simulink library "limblab"  (Simulink 6.6)
undefined symbols (not defined in the file or in its folder): dfilt
libraries: simulink x20, xpclib x10, xpcnilib x5, limblab x5, dsparch4 x4, xpcmeasurementcomputinglib x2, dspmtrx3 x1, simulink_extras x1
settings Model: Creator=limblab  LastModifiedBy=limblab

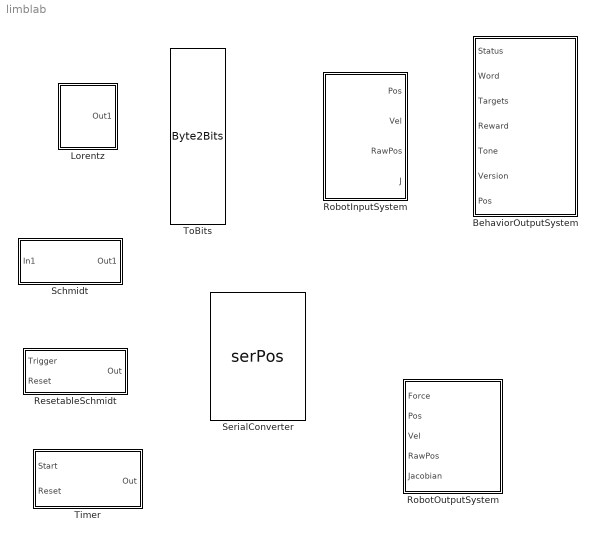
== system limblab ==
  BehaviorOutputSystem : Subsystem  TreatAsAtomicUnit=on  mask{RewardPulse=0}
      mask prompts: RewardPulse "Reward Pulse"
      mask Display:
      | port_label('input',1,'Status')
      | port_label('input',2,'Word')
      | port_label('input',3,'Targets')
      | port_label('input',4,'Reward')
      | port_label('input',5,'Tone')
      | port_label('input',6,'Version')
      | port_label('input',7,'Position')
  Lorentz : Subsystem  TreatAsAtomicUnit=on  mask(Lorentz attractor){y0=.1}
      mask prompts: y0 "Initial Condition"
      mask help: Creats chaotic oscelations using a lorentz attractor algorithm.
      mask Help:
      | Creats chaotic oscelations using a lorentz attractor algorithm.
      | 
      | This particular oscilator has the parameters:
      | rho = 28
      | beta = 8/3
      | sigma = 10
      | 
      | The initial condition y0 can be specified as a parameter.
      | 
      | Other initial conditions (x0 and z0) are 0.1.
      mask Display: port_label('output', 1, 'Out')
  ResetableSchmidt : Subsystem  TreatAsAtomicUnit=on  mask{Time=3}
  RobotInputSystem : Subsystem  TreatAsAtomicUnit=on  mask{ShOffset=0, ElOffset=0, XOffset=2, YOffset=-36, Ang=0}
      mask prompts: ShOffset "Shoulder Offset"; ElOffset "Elbow Offset"; XOffset "X Offset"; YOffset "Y Offset"; Ang "Cursor Rotation"
      mask Display:
      | port_label('output',1,'Position')
      | port_label('output',2,'Velocity')
      | port_label('output',3,'Raw Position')
      | port_label('output',4,'Jacobian')
  RobotOutputSystem : Subsystem  TreatAsAtomicUnit=on  mask{RecFlag=off, XHighLimit=25, XLowLimit=-30, YHighLimit=-46, YLowLimit=-22}
      mask prompts: RecFlag "Recenter Handle"; XHighLimit "X Upper Limit"; XLowLimit "X Lower Limit"; YHighLimit "Y Upper Limit"; YLowLimit "Y Lower Limit"
      mask Display:
      | port_label('input', 1, 'Force')
      | port_label('input', 2, 'Position')
      | port_label('input', 3, 'Velocity')
      | port_label('input', 4, 'Raw Position')
      | port_label('input', 5, 'Jacobian')
  Schmidt : Subsystem  TreatAsAtomicUnit=on  mask(Schmidt Trigger){Time=.3}
      mask help: Creates an output pulse of the specified time in seconds when trig goes high
      mask Help: Creates an output pulse of the specified time in seconds when trig goes high
      mask Display:
      | port_label('output',1,'out')
      | port_label('input',1,'trig')
      | fprintf('t = %.2f',Time)
  SerialConverter : S-Function  FunctionName=serPos
      mask Display:
      | port_label('output', 1, 'Byte Out')
      | port_label('input', 1, 'index')
      | port_label('input', 2, 'sh')
      | port_label('input', 3, 'el')
  Timer : Subsystem  TreatAsAtomicUnit=on  mask{Time=.1}
      mask prompts: Time "Timeout"
      mask Display:
      | port_label('output',1,'out')
      | port_label('input',1,'start')
      | port_label('input',2,'reset')
      | fprintf('t = %.2f',Time)
  ToBits : S-Function  FunctionName=Byte2Bits
      mask Display:
      | port_label('input', 1, 'u')
      | port_label('output', 1, 'y0')
      | port_label('output', 2, 'y1')
      | port_label('output', 3, 'y2')
      | port_label('output', 4, 'y3')
      | port_label('output', 5, 'y4')
      | port_label('output', 6, 'y5')
      | port_label('output', 7, 'y6')
      | port_label('output', 8, 'y7')

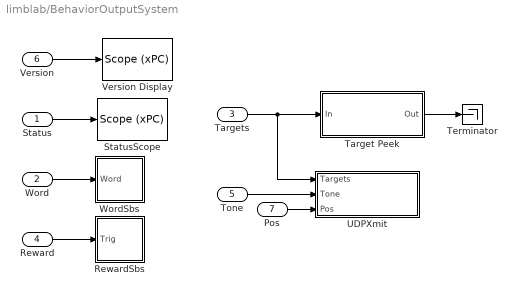
== system limblab/BehaviorOutputSystem ==
  Status : Inport
  Word : Inport  Port=2
  Targets : Inport  Port=3
  Reward : Inport  Port=4
  Tone : Inport  Port=5
  Version : Inport  Port=6
  Pos : Inport  Port=7
  RewardSbs : Subsystem
  StatusScope : xpclib/Misc./Scope (xPC)   SystemSampleTime=-1  scopeno=2  scopetype=Target  autostart=on  viewmode=Numerical  formatstr='%6.0f state,%6.0f rewards,%6.0f aborts,%6.0f fails,%6.0f incompl'  grid=on  ylimits=[-10,10]  nosamples=10  noprepostsamples=0  interleave=10  triggermode=FreeRun  triggersignal=1  triggerlevel=0.0  triggerslope=Either  triggerscope=1  triggersample=0  filename=data.dat  mode=Lazy  writesize=512  autorestart=off
  Target Peek : Subsystem
  Terminator : Terminator
  UDPXmit : Subsystem
  Version Display : xpclib/Misc./Scope (xPC)   SystemSampleTime=-1  scopeno=3  scopetype=Target  autostart=on  viewmode=Numerical  formatstr='%6.0f major,%6.0f minor,%6.0f revision,%6.0f build'  grid=on  ylimits=[-10,10]  nosamples=10  noprepostsamples=0  interleave=10  triggermode=FreeRun  triggersignal=1  triggerlevel=0.0  triggerslope=Either  triggerscope=1  triggersample=0  filename=data.dat  mode=Lazy  writesize=512  autorestart=off
  WordSbs : Subsystem
  wires:
  Status/1 -> StatusScope/1
  Word/1 -> WordSbs/1(Word)
  Targets/1 -> Target Peek/1(In), UDPXmit/1(Targets)
  Reward/1 -> RewardSbs/1(Trig)
  Target Peek/1(Out) -> Terminator/1
  Version/1 -> Version Display/1
  Pos/1 -> UDPXmit/3(Pos)
  Tone/1 -> UDPXmit/2(Tone)

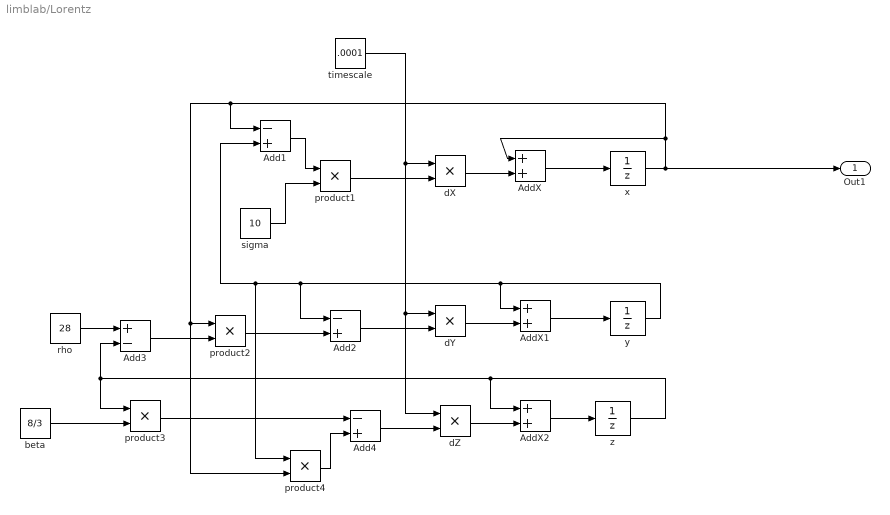
== system limblab/Lorentz ==
  Add1 : Sum  Inputs=-+  OutScaling=2^-10
  Add2 : Sum  Inputs=-+  OutScaling=2^-10
  Add3 : Sum  Inputs=+-  OutScaling=2^-10
  Add4 : Sum  Inputs=-+  OutScaling=2^-10
  AddX : Sum  OutScaling=2^-10
  AddX1 : Sum  OutScaling=2^-10
  AddX2 : Sum  OutScaling=2^-10
  beta : Constant  Value=8/3
  dX : Product  RndMeth=Zero
  dY : Product  RndMeth=Zero
  dZ : Product  RndMeth=Zero
  product{1..4} (4 alike) : Product  RndMeth=Zero
  rho : Constant  Value=28
  sigma : Constant  Value=10
  timescale : Constant  Value=.0001
  x : UnitDelay  X0=.1  SampleTime=.001
  y : UnitDelay  X0=y0  SampleTime=.001
  z : UnitDelay  X0=.1  SampleTime=.001
  Out1 : Outport
  wires:
  AddX/1 -> x/1
  AddX1/1 -> y/1
  AddX2/1 -> z/1
  y/1 -> AddX1/1, Add2/1, Add1/2, product4/1
  z/1 -> AddX2/1, Add3/2, product3/1
  x/1 -> Out1/1, AddX/1, Add1/1, product2/1, product4/2
  dX/1 -> AddX/2
  dY/1 -> AddX1/2
  dZ/1 -> AddX2/2
  timescale/1 -> dX/1, dY/1, dZ/1
  sigma/1 -> product1/2
  product1/1 -> dX/2
  Add1/1 -> product1/1
  Add2/1 -> dY/2
  product2/1 -> Add2/2
  Add3/1 -> product2/2
  rho/1 -> Add3/1
  beta/1 -> product3/2
  product3/1 -> Add4/1
  product4/1 -> Add4/2
  Add4/1 -> dZ/2

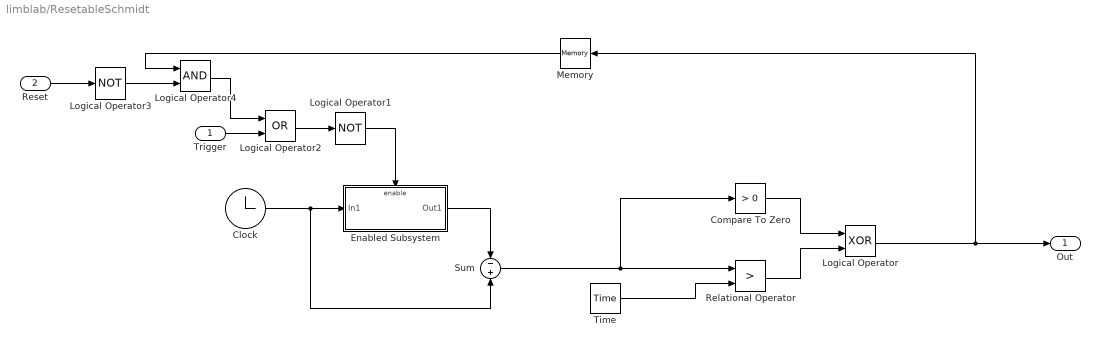
== system limblab/ResetableSchmidt ==
  Trigger : Inport
  Reset : Inport  Port=2
  Clock : Clock
  Compare To Zero : simulink/Logic and Bit Operations/Compare To Zero  SystemSampleTime=-1  relop=>  LogicOutDataTypeMode=uint8  ZeroCross=off
  Enabled Subsystem : Subsystem  TreatAsAtomicUnit=on
  Logical Operator : Logic  Operator=XOR  AllPortsSameDT=off  OutDataTypeMode=Boolean  SampleTime=.001
  Logical Operator1 : Logic  Operator=NOT  AllPortsSameDT=off  OutDataTypeMode=Boolean
  Logical Operator2 : Logic  Operator=OR  AllPortsSameDT=off  OutDataTypeMode=Boolean  SampleTime=.001
  Logical Operator3 : Logic  Operator=NOT  AllPortsSameDT=off  OutDataTypeMode=Boolean
  Logical Operator4 : Logic  AllPortsSameDT=off  OutDataTypeMode=Boolean  SampleTime=.001
  Memory : Memory  Orientation=left
  Relational Operator : RelationalOperator  Operator=>  LogicOutDataTypeMode=Boolean
  Sum : Sum  Inputs=-+
  Time : Constant  Value=Time
  Out : Outport
  wires:
  Logical Operator2/1 -> Logical Operator1/1
  Trigger/1 -> Logical Operator2/2
  Logical Operator/1 -> Memory/1, Out/1
  Logical Operator1/1 -> Enabled Subsystem/Enable
  Relational Operator/1 -> Logical Operator/2
  Compare To Zero/1 -> Logical Operator/1
  Time/1 -> Relational Operator/2
  Sum/1 -> Relational Operator/1, Compare To Zero/1
  Enabled Subsystem/1(Out1) -> Sum/1
  Clock/1 -> Sum/2, Enabled Subsystem/1(In1)
  Reset/1 -> Logical Operator3/1
  Logical Operator3/1 -> Logical Operator4/2
  Logical Operator4/1 -> Logical Operator2/1
  Memory/1 -> Logical Operator4/1

== system limblab/RobotInputSystem ==
  Matrix Concatenation1 : Concatenate  Mode=Vector
  Velocity Calculation : Subsystem
  XY Position Subsystem : Subsystem
  Xpos : xpclib/Misc./Scope (xPC)   SystemSampleTime=-1  scopeno=1  scopetype=Target  autostart=on  viewmode=Numerical  formatstr='%15.2f X,%15.2f Y,%15.2f dX,%15.2f dY,%15.2f Fx,%15.2f Fy'  grid=on  ylimits=[-10,10]  nosamples=10  noprepostsamples=0  interleave=10  triggermode=FreeRun  triggersignal=1  triggerlevel=0.0  triggerslope=Either  triggerscope=1  triggersample=0  filename=data.dat  mode=Lazy  writesize=512  autorestart=off
  Pos : Outport
  Vel : Outport  Port=2
  RawPos : Outport  Port=3
  J : Outport  Port=4
  wires:
  Velocity Calculation/1(Vel) -> Matrix Concatenation1/2, Vel/1
  XY Position Subsystem/1(Pos) -> Velocity Calculation/1(Pos), Matrix Concatenation1/1, Pos/1
  Matrix Concatenation1/1 -> Xpos/1
  XY Position Subsystem/3(RawPos) -> RawPos/1
  XY Position Subsystem/2(J) -> Velocity Calculation/2(J), J/1

== system limblab/RobotOutputSystem ==
  Force : Inport
  Pos : Inport  Port=2
  Vel : Inport  Port=3
  RawPos : Inport  Port=4
  Jacobian : Inport  Port=5
  BoundingBox : Subsystem
  Motor Control : Subsystem
  Recentering Subsystem : Subsystem
  wires:
  Recentering Subsystem/2(toSwitch) -> Motor Control/3(Switch)
  Recentering Subsystem/1(Forces) -> Motor Control/2(Recenter/Arrest Force)
  BoundingBox/1(Out) -> Recentering Subsystem/3(OutsideBox)
  Force/1 -> Motor Control/1(DefaultForce)
  Jacobian/1 -> Motor Control/4(Jacobian)
  Vel/1 -> Recentering Subsystem/1(Vel)
  Pos/1 -> Recentering Subsystem/2(Pos)
  RawPos/1 -> BoundingBox/1(RawPos)

== system limblab/Schmidt ==
  In1 : Inport
  Clock : Clock
  Compare To Zero : simulink/Logic and Bit Operations/Compare To Zero  SystemSampleTime=-1  relop=>  LogicOutDataTypeMode=uint8  ZeroCross=off
  Enabled Subsystem : Subsystem  TreatAsAtomicUnit=on
  Logical Operator : Logic  Operator=XOR  AllPortsSameDT=off  OutDataTypeMode=Boolean  SampleTime=.001
  Logical Operator1 : Logic  Operator=NOT  AllPortsSameDT=off  OutDataTypeMode=Boolean
  Logical Operator2 : Logic  Operator=OR  AllPortsSameDT=off  OutDataTypeMode=Boolean  SampleTime=.001
  Memory : Memory  Orientation=left
  Relational Operator : RelationalOperator  Operator=>  LogicOutDataTypeMode=Boolean
  Sum : Sum  Inputs=-+
  Time : Constant  Value=Time
  Out1 : Outport
  wires:
  Clock/1 -> Enabled Subsystem/1(In1), Sum/2
  Enabled Subsystem/1(Out1) -> Sum/1
  Sum/1 -> Compare To Zero/1, Relational Operator/1
  Time/1 -> Relational Operator/2
  Compare To Zero/1 -> Logical Operator/1
  Relational Operator/1 -> Logical Operator/2
  Logical Operator1/1 -> Enabled Subsystem/Enable
  Logical Operator/1 -> Out1/1, Memory/1
  In1/1 -> Logical Operator2/2
  Logical Operator2/1 -> Logical Operator1/1
  Memory/1 -> Logical Operator2/1

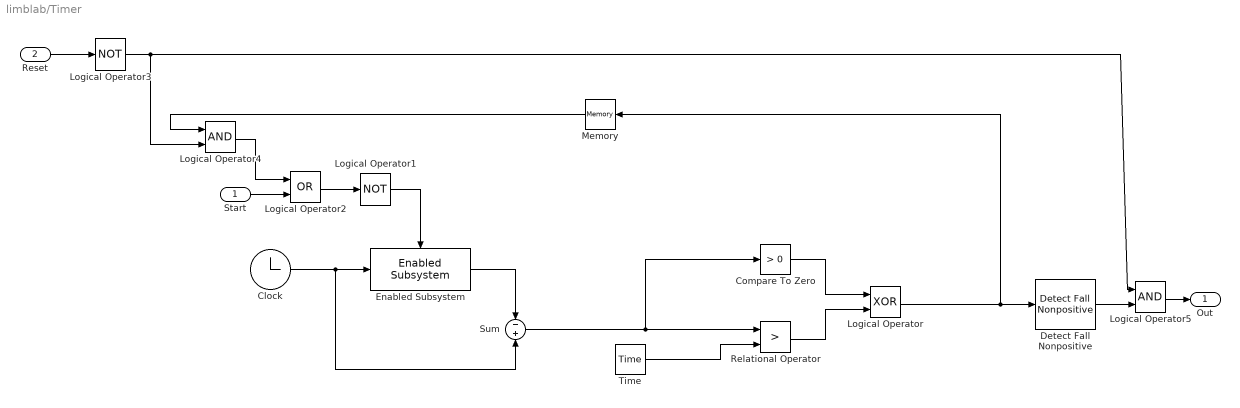
== system limblab/Timer ==
  Start : Inport
  Reset : Inport  Port=2
  Clock : Clock
  Compare To Zero : simulink/Logic and Bit Operations/Compare To Zero  SystemSampleTime=-1  relop=>  LogicOutDataTypeMode=uint8  ZeroCross=off
  Detect Fall Nonpositive : simulink/Logic and Bit Operations/Detect Fall Nonpositive  SystemSampleTime=-1  vinit=0
  Enabled Subsystem : limblab/ResetableSchmidt/Enabled Subsystem  SystemSampleTime=-1
  Logical Operator : Logic  Operator=XOR  AllPortsSameDT=off  OutDataTypeMode=Boolean  SampleTime=.001
  Logical Operator1 : Logic  Operator=NOT  AllPortsSameDT=off  OutDataTypeMode=Boolean
  Logical Operator2 : Logic  Operator=OR  AllPortsSameDT=off  OutDataTypeMode=Boolean  SampleTime=.001
  Logical Operator3 : Logic  Operator=NOT  AllPortsSameDT=off  OutDataTypeMode=Boolean
  Logical Operator4 : Logic  AllPortsSameDT=off  OutDataTypeMode=Boolean  SampleTime=.001
  Logical Operator5 : Logic  AllPortsSameDT=off  OutDataTypeMode=Boolean  SampleTime=.001
  Memory : Memory  Orientation=left
  Relational Operator : RelationalOperator  Operator=>  LogicOutDataTypeMode=Boolean
  Sum : Sum  Inputs=-+
  Time : Constant  Value=Time
  Out : Outport
  wires:
  Memory/1 -> Logical Operator4/1
  Logical Operator4/1 -> Logical Operator2/1
  Logical Operator3/1 -> Logical Operator5/1, Logical Operator4/2
  Reset/1 -> Logical Operator3/1
  Clock/1 -> Sum/2, Enabled Subsystem/1
  Enabled Subsystem/1 -> Sum/1
  Sum/1 -> Relational Operator/1, Compare To Zero/1
  Time/1 -> Relational Operator/2
  Compare To Zero/1 -> Logical Operator/1
  Relational Operator/1 -> Logical Operator/2
  Logical Operator1/1 -> Enabled Subsystem/Enable
  Logical Operator/1 -> Memory/1, Detect Fall Nonpositive/1
  Start/1 -> Logical Operator2/2
  Logical Operator2/1 -> Logical Operator1/1
  Detect Fall Nonpositive/1 -> Logical Operator5/2
  Logical Operator5/1 -> Out/1

== system limblab/BehaviorOutputSystem/RewardSbs ==
  Trig : Inport
  Data Type Conversion : DataTypeConversion
  Memory1 : Memory
  Schmidt1 : Subsystem  mask(Schmidt Trigger){Time=RewardPulse}
      mask help: Creates an output pulse of the specified time in seconds when trig goes high
      mask Help: Creates an output pulse of the specified time in seconds when trig goes high
      mask Display:
      | port_label('output',1,'out')
      | port_label('input',1,'trig')
      | fprintf('t = %.2f',Time)
  tag scope: Reward=global
  wires:
  Trig/1 -> Schmidt1/1(In1)
  Schmidt1/1(Out1) -> Memory1/1
  Memory1/1 -> Data Type Conversion/1
  Data Type Conversion/1 -> [Reward]

== system limblab/BehaviorOutputSystem/Target Peek ==
  In : Inport
  Add : Sum  OutScaling=2^-10
  Add1 : Sum  OutScaling=2^-10
  Demux : Demux  Outputs=10
  Gain : Gain  Gain=.5
  Gain1 : Gain  Gain=.5
  Mux : Mux  Inputs=3
  Terminator{,1..4} (5 alike) : Terminator
  Out : Outport
  wires:
  In/1 -> Demux/1
  Mux/1 -> Out/1
  Demux/1 -> Mux/1
  Add/1 -> Gain/1
  Add1/1 -> Gain1/1
  Gain1/1 -> Mux/3
  Demux/7 -> Terminator/1
  Demux/8 -> Terminator1/1
  Demux/9 -> Terminator2/1
  Demux/10 -> Terminator3/1
  Demux/2 -> Add/1
  Demux/4 -> Add/2
  Demux/3 -> Add1/1
  Demux/5 -> Add1/2
  Demux/6 -> Terminator4/1
  Gain/1 -> Mux/2

== system limblab/BehaviorOutputSystem/UDPXmit ==
  Targets : Inport
  Tone : Inport  Port=2
  Pos : Inport  Port=3
  Demux : Demux  Outputs=10
  Demux1 : Demux  Outputs=2
  Demux2 : Demux  Outputs=2
  Pack : xpclib/UDP/Pack  datatypes={'double', 'double','double','double','double','double','double','double','double','double','double','double','double','double'}  byteAlign=1
  Rate Transition : RateTransition
  Send : xpclib/UDP/Send  ipAddress=192.168.0.2  ipPort=25000  localPort=-1  sampletime=.02
  wires:
  Rate Transition/1 -> Send/1
  Pack/1 -> Rate Transition/1
  Demux/10 -> Pack/12
  Demux/9 -> Pack/11
  Demux/8 -> Pack/10
  Demux/7 -> Pack/9
  Demux/6 -> Pack/8
  Demux/5 -> Pack/7
  Demux/4 -> Pack/6
  Demux/3 -> Pack/5
  Demux/2 -> Pack/4
  Demux/1 -> Pack/3
  Demux1/1 -> Pack/1
  Demux1/2 -> Pack/2
  Demux2/1 -> Pack/13
  Demux2/2 -> Pack/14
  Tone/1 -> Demux2/1
  Targets/1 -> Demux/1
  Pos/1 -> Demux1/1

== system limblab/BehaviorOutputSystem/WordSbs ==
  Word : Inport
  tag scope: Word=global
  wires:
  Word/1 -> [Word]

== system limblab/ResetableSchmidt/Enabled Subsystem ==
  In1 : Inport
  Enable : EnablePort
  Out1 : Outport
  wires:
  In1/1 -> Out1/1

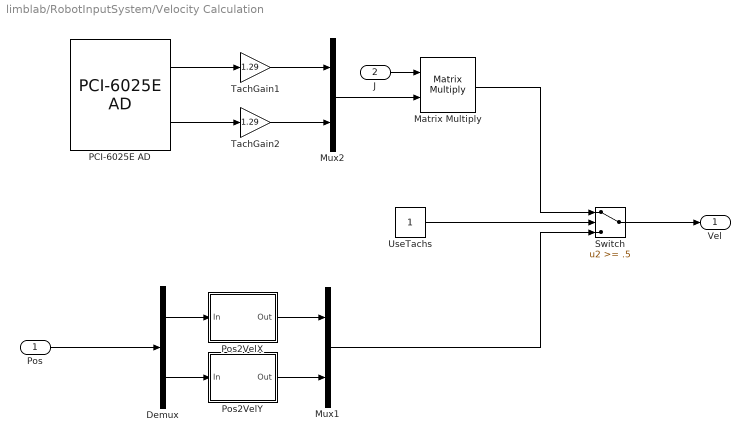
== system limblab/RobotInputSystem/Velocity Calculation ==
  Pos : Inport
  J : Inport  Port=2
  Demux : Demux  Outputs=2
  Matrix Multiply : Product  Multiplication=Matrix(*)
  Mux1 : Mux  Inputs=2
  Mux2 : Mux  Inputs=2
  PCI-6025E AD : xpcnilib/A//D/PCI-6025E AD  channel=[1,2]  range=[-10,-10]  coupling=[0,0]  sampletime=0.001  slot=-1
  Pos2VelX : Subsystem
  Pos2VelY : Subsystem
  Switch : Switch  Threshold=.5
  TachGain1 : Gain  Gain=1.29
  TachGain2 : Gain  Gain=1.29
  UseTachs : Constant
  Vel : Outport
  wires:
  Pos2VelX/1(Out) -> Mux1/1
  Pos2VelY/1(Out) -> Mux1/2
  Demux/1 -> Pos2VelX/1(In)
  Demux/2 -> Pos2VelY/1(In)
  Pos/1 -> Demux/1
  UseTachs/1 -> Switch/2
  PCI-6025E AD/1 -> TachGain1/1
  PCI-6025E AD/2 -> TachGain2/1
  TachGain1/1 -> Mux2/1
  TachGain2/1 -> Mux2/2
  J/1 -> Matrix Multiply/1
  Mux2/1 -> Matrix Multiply/2
  Switch/1 -> Vel/1
  Mux1/1 -> Switch/3
  Matrix Multiply/1 -> Switch/1

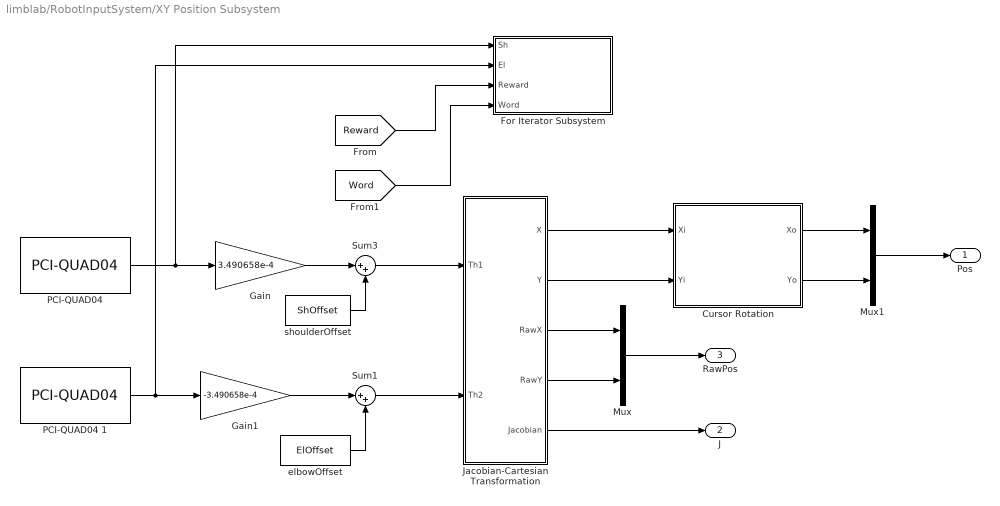
== system limblab/RobotInputSystem/XY Position Subsystem ==
  Cursor Rotation : Subsystem
  For Iterator Subsystem : Subsystem  TreatAsAtomicUnit=on
  Gain : Gain  Gain=3.490658e-4
  Gain1 : Gain  Gain=-3.490658e-4
  Jacobian-Cartesian Transformation : Subsystem
  Mux : Mux  Inputs=2
  Mux1 : Mux  Inputs=2
  "PCI-QUAD04 " : xpcmeasurementcomputinglib/Incremental Encoder/PCI-QUAD04   channel=1  resetmode=on  polarity=Positive Index  mode=Normal  limit=0  range=-2^23...+2^23-1  speed=1x  prescale=0  ts=0.001  convbaseaddr=-1
  PCI-QUAD04 1 : xpcmeasurementcomputinglib/Incremental Encoder/PCI-QUAD04   channel=2  resetmode=on  polarity=Positive Index  mode=Normal  limit=0  range=-2^23...+2^23-1  speed=1x  prescale=0  ts=0.001  convbaseaddr=-1
  Sum1 : Sum  Inputs=|++  SaturateOnIntegerOverflow=on  InputSameDT=on
  Sum3 : Sum  Inputs=|++  SaturateOnIntegerOverflow=on  InputSameDT=on
  elbowOffset : Constant  Value=ElOffset
  shoulderOffset : Constant  Value=ShOffset
  Pos : Outport
  J : Outport  Port=2
  RawPos : Outport  Port=3
  wires:
  PCI-QUAD04 1/1 -> For Iterator Subsystem/2("El "), Gain1/1
  "PCI-QUAD04 "/1 -> For Iterator Subsystem/1(Sh), Gain/1
  Gain/1 -> Sum3/1
  Sum3/1 -> Jacobian-Cartesian Transformation/1(Th1)
  shoulderOffset/1 -> Sum3/2
  Gain1/1 -> Sum1/1
  elbowOffset/1 -> Sum1/2
  Sum1/1 -> Jacobian-Cartesian Transformation/2(Th2)
  Jacobian-Cartesian Transformation/1(X) -> Cursor Rotation/1(Xi)
  Jacobian-Cartesian Transformation/2(Y) -> Cursor Rotation/2(Yi)
  Cursor Rotation/1(Xo) -> Mux1/1
  Cursor Rotation/2(Yo) -> Mux1/2
  Jacobian-Cartesian Transformation/3(RawX) -> Mux/1
  Jacobian-Cartesian Transformation/4(RawY) -> Mux/2
  [Reward] -> For Iterator Subsystem/3(Reward)
  Jacobian-Cartesian Transformation/5(Jacobian) -> J/1
  Mux/1 -> RawPos/1
  Mux1/1 -> Pos/1
  [Word] -> For Iterator Subsystem/4(Word)

== system limblab/RobotOutputSystem/BoundingBox ==
  note: 1: if [X Y] is outside
      | bounding box
      | 0: otherwise
  RawPos : Inport
  Demux : Demux  Outputs=2
  Logical Operator : Logic  Operator=OR  Inputs=4  AllPortsSameDT=off  OutDataTypeMode=Boolean
  Relational Operator : RelationalOperator  Operator=<  LogicOutDataTypeMode=Boolean
  Relational Operator1 : RelationalOperator  Operator=>  LogicOutDataTypeMode=Boolean
  Relational Operator2 : RelationalOperator  Operator=<  LogicOutDataTypeMode=Boolean
  Relational Operator3 : RelationalOperator  Operator=>  LogicOutDataTypeMode=Boolean
  XHighLimit : Constant  Value=XHighLimit
  XLowLimit : Constant  Value=XLowLimit
  YHighLimit : Constant  Value=YHighLimit
  YLowLimit : Constant  Value=YLowLimit
  Out : Outport
  wires:
  XLowLimit/1 -> Relational Operator/2
  XHighLimit/1 -> Relational Operator1/2
  YHighLimit/1 -> Relational Operator2/2
  YLowLimit/1 -> Relational Operator3/2
  Relational Operator/1 -> Logical Operator/1
  Relational Operator1/1 -> Logical Operator/2
  Relational Operator2/1 -> Logical Operator/3
  Relational Operator3/1 -> Logical Operator/4
  Logical Operator/1 -> Out/1
  RawPos/1 -> Demux/1
  Demux/1 -> Relational Operator/1, Relational Operator1/1
  Demux/2 -> Relational Operator2/1, Relational Operator3/1

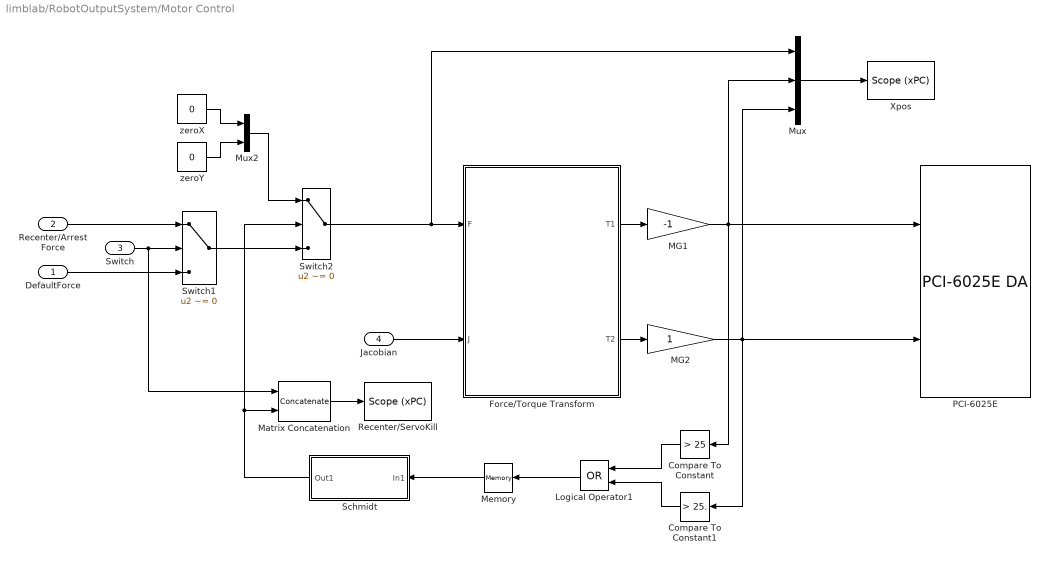
== system limblab/RobotOutputSystem/Motor Control ==
  DefaultForce : Inport
  Recenter/Arrest Force : Inport  Port=2
  Switch : Inport  Port=3
  Jacobian : Inport  Port=4
  Compare To Constant : simulink/Logic and Bit Operations/Compare To Constant  Orientation=left  SystemSampleTime=-1  relop=>  const=25  LogicOutDataTypeMode=uint8  ZeroCross=off
  Compare To Constant1 : simulink/Logic and Bit Operations/Compare To Constant  Orientation=left  SystemSampleTime=-1  relop=>  const=25.  LogicOutDataTypeMode=uint8  ZeroCross=off
  Force/Torque Transform : Subsystem  TreatAsAtomicUnit=on
  Logical Operator1 : Logic  Orientation=left  Operator=OR  AllPortsSameDT=off  OutDataTypeMode=Boolean
  MG1 : Gain  Gain=-1
  MG2 : Gain
  Matrix Concatenation : Concatenate  Mode=Vector
  Memory : Memory  Orientation=left
  Mux : Mux  Inputs=3
  Mux2 : Mux  Inputs=2
  "PCI-6025E " : xpcnilib/D//A/PCI-6025E DA  channel=[1 2]  reset=[1 1]  initValue=[0 0]  sampletime=0.001  slot=-1
  Recenter/ServoKill : xpclib/Misc./Scope (xPC)   SystemSampleTime=-1  scopeno=5  scopetype=Target  autostart=on  viewmode=Numerical  formatstr='%6.0f Control,%6.0f ServoKill'  grid=on  ylimits=[-10,10]  nosamples=10  noprepostsamples=0  interleave=10  triggermode=FreeRun  triggersignal=1  triggerlevel=0.0  triggerslope=Either  triggerscope=1  triggersample=0  filename=data.dat  mode=Lazy  writesize=512  autorestart=off
  Schmidt : Subsystem  Orientation=left  mask(Schmidt Trigger){Time=3}
      mask help: Creates an output pulse of the specified time in seconds when trig goes high
      mask Help: Creates an output pulse of the specified time in seconds when trig goes high
      mask Display:
      | port_label('output',1,'out')
      | port_label('input',1,'trig')
      | fprintf('t = %d',Time)
  Switch1 : Switch  Criteria=u2 ~= 0  ZeroCross=off
  Switch2 : Switch  Criteria=u2 ~= 0  ZeroCross=off
  Xpos : xpclib/Misc./Scope (xPC)   SystemSampleTime=-1  scopeno=6  scopetype=Target  autostart=on  viewmode=Numerical  formatstr='%15.2f Fx,%15.2f Fy,%15.2f T1,%15.2f T2'  grid=on  ylimits=[-10,10]  nosamples=10  noprepostsamples=0  interleave=10  triggermode=FreeRun  triggersignal=1  triggerlevel=0.0  triggerslope=Either  triggerscope=1  triggersample=0  filename=data.dat  mode=Lazy  writesize=512  autorestart=off
  zeroX : Constant  Value=0
  zeroY : Constant  Value=0
  wires:
  MG1/1 -> Compare To Constant/1, Mux/2, "PCI-6025E "/1
  MG2/1 -> Compare To Constant1/1, Mux/3, "PCI-6025E "/2
  Force/Torque Transform/1(T1) -> MG1/1
  Force/Torque Transform/2(T2) -> MG2/1
  zeroX/1 -> Mux2/1
  zeroY/1 -> Mux2/2
  Mux2/1 -> Switch2/1
  Switch1/1 -> Switch2/3
  Switch2/1 -> Force/Torque Transform/1(F), Mux/1
  Schmidt/1(Out1) -> Switch2/2, Matrix Concatenation/2
  Compare To Constant/1 -> Logical Operator1/1
  Compare To Constant1/1 -> Logical Operator1/2
  Memory/1 -> Schmidt/1(In1)
  Logical Operator1/1 -> Memory/1
  Matrix Concatenation/1 -> Recenter/ServoKill/1
  Jacobian/1 -> Force/Torque Transform/2(J)
  Switch/1 -> Switch1/2, Matrix Concatenation/1
  DefaultForce/1 -> Switch1/3
  Recenter/Arrest Force/1 -> Switch1/1
  Mux/1 -> Xpos/1

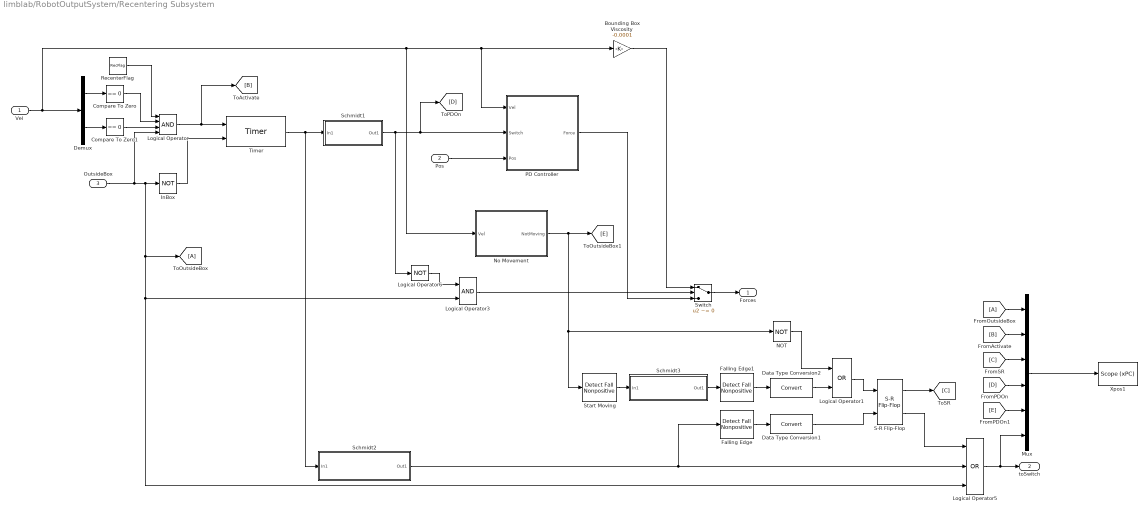
== system limblab/RobotOutputSystem/Recentering Subsystem ==
  Vel : Inport
  Pos : Inport  Port=2
  OutsideBox : Inport  Port=3
  Bounding Box Viscosity : Gain  Gain=-0.0001
  Compare To Zero : simulink/Logic and Bit Operations/Compare To Zero  SystemSampleTime=-1  relop===  LogicOutDataTypeMode=uint8  ZeroCross=off
  Compare To Zero1 : simulink/Logic and Bit Operations/Compare To Zero  SystemSampleTime=-1  relop===  LogicOutDataTypeMode=uint8  ZeroCross=off
  Data Type Conversion1 : DataTypeConversion
  Data Type Conversion2 : DataTypeConversion
  Demux : Demux  Outputs=2
  Falling Edge : simulink/Logic and Bit Operations/Detect Fall Nonpositive  SystemSampleTime=-1  vinit=0
  Falling Edge1 : simulink/Logic and Bit Operations/Detect Fall Nonpositive  SystemSampleTime=-1  vinit=0
  InBox : Logic  Operator=NOT  AllPortsSameDT=off  OutDataTypeMode=Boolean
  Logical Operator : Logic  Inputs=4  AllPortsSameDT=off  OutDataTypeMode=Boolean
  Logical Operator1 : Logic  Operator=OR  AllPortsSameDT=off  OutDataTypeMode=Boolean
  Logical Operator3 : Logic  AllPortsSameDT=off  OutDataTypeMode=Boolean
  Logical Operator5 : Logic  Operator=OR  Inputs=3  AllPortsSameDT=off  OutDataTypeMode=Boolean
  Logical Operator6 : Logic  Operator=NOT  AllPortsSameDT=off  OutDataTypeMode=Boolean
  Mux : Mux  Inputs=6
  NOT : Logic  Operator=NOT  AllPortsSameDT=off  OutDataTypeMode=Boolean  LogicDataType=double
  No Movement : Subsystem
  PD Controller : Subsystem
  RecenterFlag : Constant  Value=RecFlag
  S-R Flip-Flop : simulink_extras/Flip Flops/S-R Flip-Flop  SystemSampleTime=-1  initial_condition=0
  Schmidt1 : Subsystem  mask(Schmidt Trigger){Time=4}
      mask help: Creates an output pulse of the specified time in seconds when trig goes high
      mask Help: Creates an output pulse of the specified time in seconds when trig goes high
      mask Display:
      | port_label('output',1,'out')
      | port_label('input',1,'trig')
      | fprintf('t = %d',Time)
  Schmidt2 : Subsystem  mask(Schmidt Trigger){Time=5}
      mask help: Creates an output pulse of the specified time in seconds when trig goes high
      mask Help: Creates an output pulse of the specified time in seconds when trig goes high
      mask Display:
      | port_label('output',1,'out')
      | port_label('input',1,'trig')
      | fprintf('t = %d',Time)
  Schmidt3 : Subsystem  mask(Schmidt Trigger){Time=0.5}
      mask help: Creates an output pulse of the specified time in seconds when trig goes high
      mask Help: Creates an output pulse of the specified time in seconds when trig goes high
      mask Display:
      | port_label('output',1,'out')
      | port_label('input',1,'trig')
      | fprintf('t = %d',Time)
  Start Moving : simulink/Logic and Bit Operations/Detect Fall Nonpositive  SystemSampleTime=-1  vinit=0
  Switch : Switch  Criteria=u2 ~= 0
  Timer : limblab/Timer  SystemSampleTime=-1  Time=10
  Xpos1 : xpclib/Misc./Scope (xPC)   SystemSampleTime=-1  scopeno=4  scopetype=Target  autostart=on  viewmode=Numerical  formatstr='%2.0f OutsideBox,%2.0f Activate,%2.0f SR,%2.0f OD On,%2.0f no movement,%2.0f claimed'  grid=on  ylimits=[-10,10]  nosamples=10  noprepostsamples=0  interleave=10  triggermode=FreeRun  triggersignal=1  triggerlevel=0.0  triggerslope=Either  triggerscope=1  triggersample=0  filename=data.dat  mode=Lazy  writesize=512  autorestart=off
  Forces : Outport
  toSwitch : Outport  Port=2
  wires:
  Demux/2 -> Compare To Zero1/1
  Compare To Zero/1 -> Logical Operator/2
  Schmidt1/1(Out1) -> Logical Operator6/1, PD Controller/2(Switch), [D]
  Logical Operator/1 -> Timer/1, [B]
  OutsideBox/1 -> [A], Logical Operator3/2, Logical Operator5/3, InBox/1, Logical Operator/4
  Switch/1 -> Forces/1
  Logical Operator5/1 -> toSwitch/1, Mux/6
  Logical Operator6/1 -> Logical Operator3/1
  InBox/1 -> Timer/2
  Vel/1 -> Demux/1, No Movement/1(Vel), PD Controller/1(Vel), Bounding Box Viscosity/1
  Timer/1 -> Schmidt1/1(In1), Schmidt2/1(In1)
  Compare To Zero1/1 -> Logical Operator/3
  Demux/1 -> Compare To Zero/1
  Logical Operator3/1 -> Switch/2
  RecenterFlag/1 -> Logical Operator/1
  PD Controller/1(Force) -> Switch/3
  Pos/1 -> PD Controller/3(Pos)
  Bounding Box Viscosity/1 -> Switch/1
  Mux/1 -> Xpos1/1
  [A] -> Mux/1
  [B] -> Mux/2
  [D] -> Mux/4
  [C] -> Mux/3
  [E] -> Mux/5
  Schmidt2/1(Out1) -> Logical Operator5/2, Falling Edge/1
  S-R Flip-Flop/1 -> [C]
  S-R Flip-Flop/2 -> Logical Operator5/1
  Falling Edge/1 -> Data Type Conversion1/1
  Data Type Conversion1/1 -> S-R Flip-Flop/2
  Start Moving/1 -> Schmidt3/1(In1)
  Schmidt3/1(Out1) -> Falling Edge1/1
  Falling Edge1/1 -> Data Type Conversion2/1
  Data Type Conversion2/1 -> Logical Operator1/2
  Logical Operator1/1 -> S-R Flip-Flop/1
  No Movement/1(NotMoving) -> [E], Start Moving/1, NOT/1
  NOT/1 -> Logical Operator1/1

== system limblab/Schmidt/Enabled Subsystem ==
  In1 : Inport
  Enable : EnablePort
  Out1 : Outport
  wires:
  In1/1 -> Out1/1

== system limblab/BehaviorOutputSystem/RewardSbs/Schmidt1 ==
  In1 : Inport
  Clock : Clock
  Compare To Zero : simulink/Logic and Bit Operations/Compare To Zero  SystemSampleTime=-1  relop=>  LogicOutDataTypeMode=uint8  ZeroCross=off
  Enabled Subsystem : Subsystem  TreatAsAtomicUnit=on
  Logical Operator : Logic  Operator=XOR  AllPortsSameDT=off  OutDataTypeMode=Boolean  SampleTime=.001
  Logical Operator1 : Logic  Operator=NOT  AllPortsSameDT=off  OutDataTypeMode=Boolean
  Logical Operator2 : Logic  Operator=OR  AllPortsSameDT=off  OutDataTypeMode=Boolean  SampleTime=.001
  Memory : Memory  Orientation=left
  Relational Operator : RelationalOperator  Operator=>  LogicOutDataTypeMode=Boolean
  Sum : Sum  Inputs=-+
  Time : Constant  Value=Time
  Out1 : Outport
  wires:
  Clock/1 -> Enabled Subsystem/1(In1), Sum/2
  Enabled Subsystem/1(Out1) -> Sum/1
  Sum/1 -> Compare To Zero/1, Relational Operator/1
  Time/1 -> Relational Operator/2
  Compare To Zero/1 -> Logical Operator/1
  Relational Operator/1 -> Logical Operator/2
  Logical Operator1/1 -> Enabled Subsystem/Enable
  Logical Operator/1 -> Out1/1, Memory/1
  In1/1 -> Logical Operator2/2
  Logical Operator2/1 -> Logical Operator1/1
  Memory/1 -> Logical Operator2/1

== system limblab/RobotInputSystem/Velocity Calculation/Pos2VelX ==
  In : Inport
  Derivative : Derivative
  Digital Filter : dsparch4/Digital Filter  DialogController=dspdialog.DigitalFilter  DialogControllerArgs=DataTag0  TypePopup=FIR (all zeros)  IIRFiltStruct=Direct form II transposed  AllPoleFiltStruct=Direct form  FIRFiltStruct=Direct form  CoeffSource=Specify via dialog  NumCoeffs="[0.0144    0.0304    0.0724    0.1245    0.1668    0.1830    0.1668    0.1245    0.0724    0.0304    0.0144]"  DenCoeffs=[1 0.1]  BiQuadCoeffs=[1 0.3 0.4 1 0.1 0.2]  LatticeCoeffs=[0.2 0.4]  denIgnore=on  FiltPerSampPopup=One filter per frame  IC=0  ICnum=0  ICden=0  roundingMode=Floor  overflowMode=off  ScaleValues=1  scaleValueFracLength=14  stageInFracLength=15  stageOutFracLength=15  FilterSource=Specify via dialog  dfiltObjectName=dfilt.dffir([1 2 1])
  Digital Filter2 : dsparch4/Digital Filter  DialogController=dspdialog.DigitalFilter  DialogControllerArgs=DataTag1  TypePopup=FIR (all zeros)  IIRFiltStruct=Direct form II transposed  AllPoleFiltStruct=Direct form  FIRFiltStruct=Direct form  CoeffSource=Specify via dialog  NumCoeffs="[0.0144    0.0304    0.0724    0.1245    0.1668    0.1830    0.1668    0.1245    0.0724    0.0304    0.0144]"  DenCoeffs=[1 0.1]  BiQuadCoeffs=[1 0.3 0.4 1 0.1 0.2]  LatticeCoeffs=[0.2 0.4]  denIgnore=on  FiltPerSampPopup=One filter per frame  IC=0  ICnum=0  ICden=0  roundingMode=Floor  overflowMode=off  ScaleValues=1  scaleValueFracLength=14  stageInFracLength=15  stageOutFracLength=15  FilterSource=Specify via dialog  dfiltObjectName=dfilt.dffir([1 2 1])
  dG : Gain  SampleTime=.001
  Out : Outport
  wires:
  Derivative/1 -> dG/1
  dG/1 -> Digital Filter/1
  Digital Filter2/1 -> Derivative/1
  In/1 -> Digital Filter2/1
  Digital Filter/1 -> Out/1

== system limblab/RobotInputSystem/Velocity Calculation/Pos2VelY ==
  In : Inport
  Derivative : Derivative
  Digital Filter : dsparch4/Digital Filter  DialogController=dspdialog.DigitalFilter  DialogControllerArgs=DataTag2  TypePopup=FIR (all zeros)  IIRFiltStruct=Direct form II transposed  AllPoleFiltStruct=Direct form  FIRFiltStruct=Direct form  CoeffSource=Specify via dialog  NumCoeffs="[0.0144    0.0304    0.0724    0.1245    0.1668    0.1830    0.1668    0.1245    0.0724    0.0304    0.0144]"  DenCoeffs=[1 0.1]  BiQuadCoeffs=[1 0.3 0.4 1 0.1 0.2]  LatticeCoeffs=[0.2 0.4]  denIgnore=on  FiltPerSampPopup=One filter per frame  IC=0  ICnum=0  ICden=0  roundingMode=Floor  overflowMode=off  ScaleValues=1  scaleValueFracLength=14  stageInFracLength=15  stageOutFracLength=15  FilterSource=Specify via dialog  dfiltObjectName=dfilt.dffir([1 2 1])
  Digital Filter2 : dsparch4/Digital Filter  DialogController=dspdialog.DigitalFilter  DialogControllerArgs=DataTag3  TypePopup=FIR (all zeros)  IIRFiltStruct=Direct form II transposed  AllPoleFiltStruct=Direct form  FIRFiltStruct=Direct form  CoeffSource=Specify via dialog  NumCoeffs="[0.0144    0.0304    0.0724    0.1245    0.1668    0.1830    0.1668    0.1245    0.0724    0.0304    0.0144]"  DenCoeffs=[1 0.1]  BiQuadCoeffs=[1 0.3 0.4 1 0.1 0.2]  LatticeCoeffs=[0.2 0.4]  denIgnore=on  FiltPerSampPopup=One filter per frame  IC=0  ICnum=0  ICden=0  roundingMode=Floor  overflowMode=off  ScaleValues=1  scaleValueFracLength=14  stageInFracLength=15  stageOutFracLength=15  FilterSource=Specify via dialog  dfiltObjectName=dfilt.dffir([1 2 1])
  dG : Gain  SampleTime=.001
  Out : Outport
  wires:
  Derivative/1 -> dG/1
  dG/1 -> Digital Filter/1
  Digital Filter2/1 -> Derivative/1
  In/1 -> Digital Filter2/1
  Digital Filter/1 -> Out/1

== system limblab/RobotInputSystem/XY Position Subsystem/Cursor Rotation ==
  Xi : Inport
  Yi : Inport  Port=2
  AngleOffset : Constant  Value=Ang  SampleTime=.001
  Mux : Mux  Inputs=2
  Product : Product  RndMeth=Zero
  Product1 : Product  RndMeth=Zero
  Sum : Sum  Inputs=|++
  Trigonometric Function : Trigonometry
  Trigonometric Function1 : Trigonometry  Operator=atan2
  Trigonometric Function2 : Trigonometry  Operator=cos
  sqrt(u[1]*u[1] + u[2]*u[2]) : Fcn  Expr=sqrt(u[1]*u[1] + u[2]*u[2])
  Xo : Outport
  Yo : Outport  Port=2
  wires:
  AngleOffset/1 -> Sum/2
  Trigonometric Function1/1 -> Sum/1
  Yi/1 -> Trigonometric Function1/1, Mux/1
  Xi/1 -> Trigonometric Function1/2, Mux/2
  Mux/1 -> sqrt(u[1]*u[1] + u[2]*u[2])/1
  Trigonometric Function/1 -> Product/2
  Product/1 -> Yo/1
  sqrt(u[1]*u[1] + u[2]*u[2])/1 -> Product/1, Product1/2
  Sum/1 -> Trigonometric Function/1, Trigonometric Function2/1
  Product1/1 -> Xo/1
  Trigonometric Function2/1 -> Product1/1

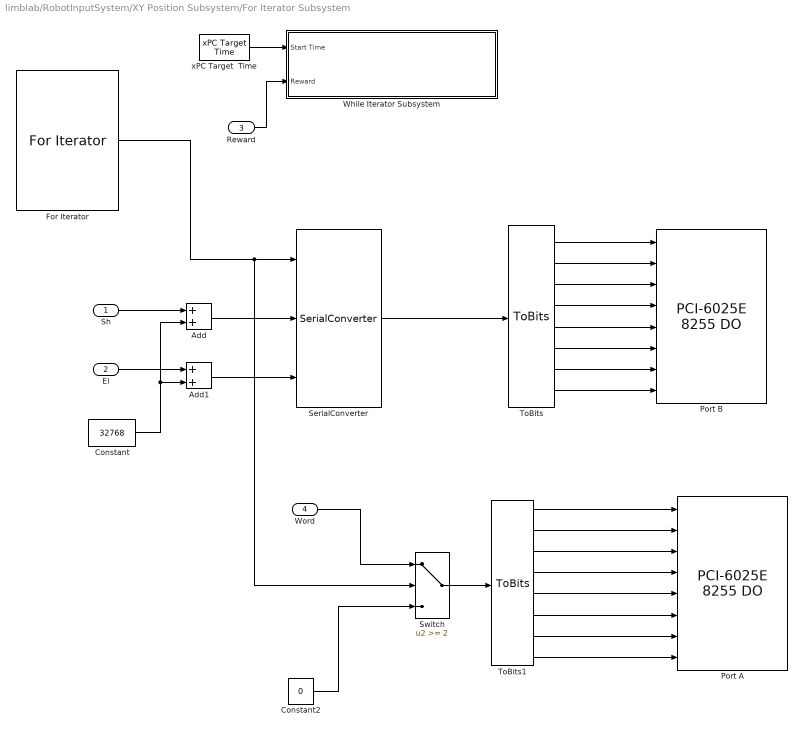
== system limblab/RobotInputSystem/XY Position Subsystem/For Iterator Subsystem ==
  Sh : Inport
  "El " : Inport  Port=2
  Reward : Inport  Port=3
  Word : Inport  Port=4
  Add : Sum  OutScaling=2^-10
  Add1 : Sum  OutScaling=2^-10
  Constant : Constant  Value=32768
  Constant2 : Constant  Value=0
  For Iterator : ForIterator  IterationLimit=4  IndexMode=Zero-based  IterationVariableDataType=double
  Port A : xpcnilib/Digital Output/PCI-6025E 8255 DO  channel=1:8  port=A  reset=[1]  initValue=[0]  chip=1  sampletime=-1  slot=-1
  Port B : xpcnilib/Digital Output/PCI-6025E 8255 DO  channel=1:8  port=B  reset=[1]  initValue=[0]  chip=1  sampletime=-1  slot=-1
  SerialConverter : limblab/SerialConverter
  Switch : Switch  Threshold=2
  ToBits : limblab/ToBits
  ToBits1 : limblab/ToBits
  While Iterator Subsystem : Subsystem  TreatAsAtomicUnit=on
  "xPC Target  Time " : xpclib/Misc./xPC Target  Time   ts=-1
  wires:
  "xPC Target  Time "/1 -> While Iterator Subsystem/1(Start Time)
  SerialConverter/1 -> ToBits/1
  For Iterator/1 -> SerialConverter/1, Switch/2
  Sh/1 -> Add/1
  Add/1 -> SerialConverter/2
  Add1/1 -> SerialConverter/3
  "El "/1 -> Add1/1
  Constant/1 -> Add/2, Add1/2
  ToBits/1 -> Port B/1
  ToBits/2 -> Port B/2
  ToBits/3 -> Port B/3
  ToBits/4 -> Port B/4
  ToBits/5 -> Port B/5
  ToBits/6 -> Port B/6
  ToBits/7 -> Port B/7
  ToBits/8 -> Port B/8
  Reward/1 -> While Iterator Subsystem/2(Reward)
  ToBits1/1 -> Port A/1
  ToBits1/2 -> Port A/2
  ToBits1/3 -> Port A/3
  ToBits1/4 -> Port A/4
  ToBits1/5 -> Port A/5
  ToBits1/6 -> Port A/6
  ToBits1/7 -> Port A/7
  ToBits1/8 -> Port A/8
  Constant2/1 -> Switch/3
  Word/1 -> Switch/1
  Switch/1 -> ToBits1/1

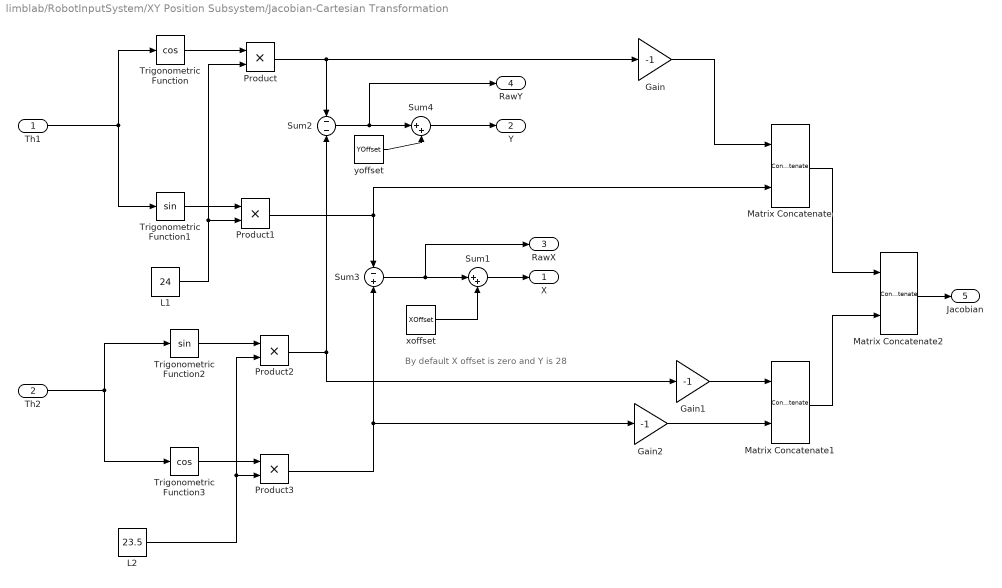
== system limblab/RobotInputSystem/XY Position Subsystem/Jacobian-Cartesian Transformation ==
  note: By default X offset is zero and Y is 28
  Th1 : Inport
  Th2 : Inport  Port=2
  Gain : Gain  Gain=-1
  Gain1 : Gain  Gain=-1
  Gain2 : Gain  Gain=-1
  L1 : Constant  Value=24
  L2 : Constant  Value=23.5
  Matrix Concatenate : Concatenate  Mode=Vector  ConcatenateDimension=2
  Matrix Concatenate1 : Concatenate  Mode=Vector  ConcatenateDimension=2
  Matrix Concatenate2 : Concatenate  Mode=Multidimensional array  ConcatenateDimension=2
  Product{,1..3} (4 alike) : Product  RndMeth=Zero
  Sum1 : Sum  Inputs=|++  SaturateOnIntegerOverflow=on  InputSameDT=on
  Sum2 : Sum  Inputs=--  SaturateOnIntegerOverflow=on  InputSameDT=on
  Sum3 : Sum  Inputs=-+  SaturateOnIntegerOverflow=on  InputSameDT=on
  Sum4 : Sum  Inputs=|++  SaturateOnIntegerOverflow=on  InputSameDT=on
  Trigonometric Function : Trigonometry  Operator=cos
  Trigonometric Function1 : Trigonometry
  Trigonometric Function2 : Trigonometry
  Trigonometric Function3 : Trigonometry  Operator=cos
  xoffset : Constant  Value=XOffset
  yoffset : Constant  Value=YOffset
  X : Outport
  Y : Outport  Port=2
  RawX : Outport  Port=3
  RawY : Outport  Port=4
  Jacobian : Outport  Port=5
  wires:
  Th1/1 -> Trigonometric Function1/1, Trigonometric Function/1
  Product/1 -> Sum2/1, Gain/1
  Product2/1 -> Sum2/2, Gain1/1
  Sum3/1 -> Sum1/1, RawX/1
  Product1/1 -> Sum3/1, Matrix Concatenate/2
  Sum2/1 -> Sum4/1, RawY/1
  Sum4/1 -> Y/1
  Sum1/1 -> X/1
  xoffset/1 -> Sum1/2
  yoffset/1 -> Sum4/2
  Product3/1 -> Sum3/2, Gain2/1
  Th2/1 -> Trigonometric Function2/1, Trigonometric Function3/1
  Matrix Concatenate/1 -> Matrix Concatenate2/1
  Matrix Concatenate1/1 -> Matrix Concatenate2/2
  Matrix Concatenate2/1 -> Jacobian/1
  Gain/1 -> Matrix Concatenate/1
  Gain1/1 -> Matrix Concatenate1/1
  Gain2/1 -> Matrix Concatenate1/2
  Trigonometric Function/1 -> Product/1
  Trigonometric Function3/1 -> Product3/1
  Trigonometric Function2/1 -> Product2/1
  L2/1 -> Product2/2, Product3/2
  Trigonometric Function1/1 -> Product1/1
  L1/1 -> Product/2, Product1/2

== system limblab/RobotOutputSystem/Motor Control/Force/Torque Transform ==
  F : Inport
  J : Inport  Port=2
  Demux2 : Demux  Outputs=2
  Gain : Gain  Gain=-1
  Matrix Multiply : Product  Multiplication=Matrix(*)
  Transpose : dspmtrx3/Transpose  SystemSampleTime=-1  Hermitian=off  overflowFlag=off
  T1 : Outport
  T2 : Outport  Port=2
  wires:
  J/1 -> Transpose/1
  Transpose/1 -> Matrix Multiply/1
  Matrix Multiply/1 -> Demux2/1
  Demux2/2 -> T2/1
  Demux2/1 -> T1/1
  Gain/1 -> Matrix Multiply/2
  F/1 -> Gain/1

== system limblab/RobotOutputSystem/Motor Control/Schmidt ==
  In1 : Inport
  Clock : Clock
  Compare To Zero : simulink/Logic and Bit Operations/Compare To Zero  SystemSampleTime=-1  relop=>  LogicOutDataTypeMode=uint8  ZeroCross=off
  Enabled Subsystem : Subsystem  TreatAsAtomicUnit=on
  Logical Operator : Logic  Operator=XOR  AllPortsSameDT=off  OutDataTypeMode=Boolean  SampleTime=.001
  Logical Operator1 : Logic  Operator=NOT  AllPortsSameDT=off  OutDataTypeMode=Boolean
  Logical Operator2 : Logic  Operator=OR  AllPortsSameDT=off  OutDataTypeMode=Boolean  SampleTime=.001
  Memory : Memory  Orientation=left
  Relational Operator : RelationalOperator  Operator=>  LogicOutDataTypeMode=Boolean
  Sum : Sum  Inputs=-+
  Time : Constant  Value=Time
  Out1 : Outport
  wires:
  Clock/1 -> Enabled Subsystem/1(In1), Sum/2
  Enabled Subsystem/1(Out1) -> Sum/1
  Sum/1 -> Compare To Zero/1, Relational Operator/1
  Time/1 -> Relational Operator/2
  Compare To Zero/1 -> Logical Operator/1
  Relational Operator/1 -> Logical Operator/2
  Logical Operator1/1 -> Enabled Subsystem/Enable
  Logical Operator/1 -> Out1/1, Memory/1
  In1/1 -> Logical Operator2/2
  Logical Operator2/1 -> Logical Operator1/1
  Memory/1 -> Logical Operator2/1

== system limblab/RobotOutputSystem/Recentering Subsystem/No Movement ==
  Vel : Inport
  Abs2 : Abs
  Abs3 : Abs
  Compare To Constant2 : simulink/Logic and Bit Operations/Compare To Constant  SystemSampleTime=-1  relop=<=  const=0.004  LogicOutDataTypeMode=uint8  ZeroCross=off
  Compare To Constant3 : simulink/Logic and Bit Operations/Compare To Constant  SystemSampleTime=-1  relop=<=  const=.004  LogicOutDataTypeMode=uint8  ZeroCross=off
  Demux1 : Demux  Outputs=2
  Logical Operator1 : Logic  AllPortsSameDT=off  OutDataTypeMode=Boolean  LogicDataType=double
  NotMoving : Outport
  wires:
  Abs2/1 -> Compare To Constant2/1
  Abs3/1 -> Compare To Constant3/1
  Logical Operator1/1 -> NotMoving/1
  Vel/1 -> Demux1/1
  Demux1/1 -> Abs2/1
  Demux1/2 -> Abs3/1
  Compare To Constant2/1 -> Logical Operator1/1
  Compare To Constant3/1 -> Logical Operator1/2

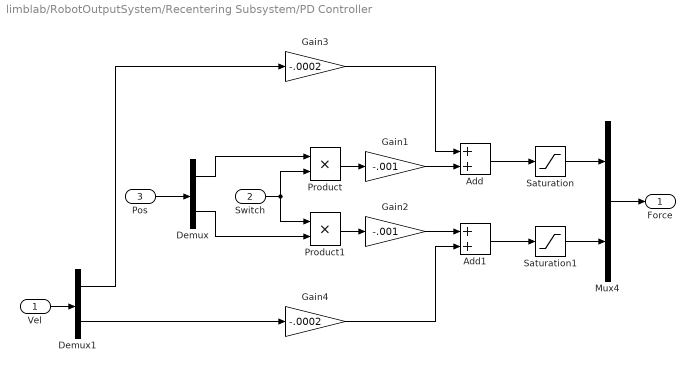
== system limblab/RobotOutputSystem/Recentering Subsystem/PD Controller ==
  Vel : Inport
  Switch : Inport  Port=2
  Pos : Inport  Port=3
  Add : Sum  OutScaling=2^-10
  Add1 : Sum  OutScaling=2^-10
  Demux : Demux  Outputs=2
  Demux1 : Demux  Outputs=2
  Gain1 : Gain  Gain=-.001
  Gain2 : Gain  Gain=-.001
  Gain3 : Gain  Gain=-.0002
  Gain4 : Gain  Gain=-.0002
  Mux4 : Mux  Inputs=2
  Product : Product  RndMeth=Zero
  Product1 : Product  RndMeth=Zero
  Saturation : Saturate  UpperLimit=.01  LowerLimit=-0.01
  Saturation1 : Saturate  UpperLimit=.01  LowerLimit=-0.01
  Force : Outport
  wires:
  Switch/1 -> Product/2, Product1/1
  Product/1 -> Gain1/1
  Saturation/1 -> Mux4/1
  Add/1 -> Saturation/1
  Gain1/1 -> Add/2
  Gain3/1 -> Add/1
  Product1/1 -> Gain2/1
  Saturation1/1 -> Mux4/2
  Add1/1 -> Saturation1/1
  Gain2/1 -> Add1/1
  Gain4/1 -> Add1/2
  Mux4/1 -> Force/1
  Demux/1 -> Product/1
  Demux/2 -> Product1/2
  Pos/1 -> Demux/1
  Vel/1 -> Demux1/1
  Demux1/2 -> Gain4/1
  Demux1/1 -> Gain3/1

== system limblab/RobotOutputSystem/Recentering Subsystem/Schmidt1 ==
  In1 : Inport
  Clock : Clock
  Compare To Zero : simulink/Logic and Bit Operations/Compare To Zero  SystemSampleTime=-1  relop=>  LogicOutDataTypeMode=uint8  ZeroCross=off
  Enabled Subsystem : Subsystem  TreatAsAtomicUnit=on
  Logical Operator : Logic  Operator=XOR  AllPortsSameDT=off  OutDataTypeMode=Boolean  SampleTime=.001
  Logical Operator1 : Logic  Operator=NOT  AllPortsSameDT=off  OutDataTypeMode=Boolean
  Logical Operator2 : Logic  Operator=OR  AllPortsSameDT=off  OutDataTypeMode=Boolean  SampleTime=.001
  Memory : Memory  Orientation=left
  Relational Operator : RelationalOperator  Operator=>  LogicOutDataTypeMode=Boolean
  Sum : Sum  Inputs=-+
  Time : Constant  Value=Time
  Out1 : Outport
  wires:
  Clock/1 -> Enabled Subsystem/1(In1), Sum/2
  Enabled Subsystem/1(Out1) -> Sum/1
  Sum/1 -> Compare To Zero/1, Relational Operator/1
  Time/1 -> Relational Operator/2
  Compare To Zero/1 -> Logical Operator/1
  Relational Operator/1 -> Logical Operator/2
  Logical Operator1/1 -> Enabled Subsystem/Enable
  Logical Operator/1 -> Out1/1, Memory/1
  In1/1 -> Logical Operator2/2
  Logical Operator2/1 -> Logical Operator1/1
  Memory/1 -> Logical Operator2/1

== system limblab/RobotOutputSystem/Recentering Subsystem/Schmidt2 ==
  In1 : Inport
  Clock : Clock
  Compare To Zero : simulink/Logic and Bit Operations/Compare To Zero  SystemSampleTime=-1  relop=>  LogicOutDataTypeMode=uint8  ZeroCross=off
  Enabled Subsystem : Subsystem  TreatAsAtomicUnit=on
  Logical Operator : Logic  Operator=XOR  AllPortsSameDT=off  OutDataTypeMode=Boolean  SampleTime=.001
  Logical Operator1 : Logic  Operator=NOT  AllPortsSameDT=off  OutDataTypeMode=Boolean
  Logical Operator2 : Logic  Operator=OR  AllPortsSameDT=off  OutDataTypeMode=Boolean  SampleTime=.001
  Memory : Memory  Orientation=left
  Relational Operator : RelationalOperator  Operator=>  LogicOutDataTypeMode=Boolean
  Sum : Sum  Inputs=-+
  Time : Constant  Value=Time
  Out1 : Outport
  wires:
  Clock/1 -> Enabled Subsystem/1(In1), Sum/2
  Enabled Subsystem/1(Out1) -> Sum/1
  Sum/1 -> Compare To Zero/1, Relational Operator/1
  Time/1 -> Relational Operator/2
  Compare To Zero/1 -> Logical Operator/1
  Relational Operator/1 -> Logical Operator/2
  Logical Operator1/1 -> Enabled Subsystem/Enable
  Logical Operator/1 -> Out1/1, Memory/1
  In1/1 -> Logical Operator2/2
  Logical Operator2/1 -> Logical Operator1/1
  Memory/1 -> Logical Operator2/1

== system limblab/RobotOutputSystem/Recentering Subsystem/Schmidt3 ==
  In1 : Inport
  Clock : Clock
  Compare To Zero : simulink/Logic and Bit Operations/Compare To Zero  SystemSampleTime=-1  relop=>  LogicOutDataTypeMode=uint8  ZeroCross=off
  Enabled Subsystem : Subsystem  TreatAsAtomicUnit=on
  Logical Operator : Logic  Operator=XOR  AllPortsSameDT=off  OutDataTypeMode=Boolean  SampleTime=.001
  Logical Operator1 : Logic  Operator=NOT  AllPortsSameDT=off  OutDataTypeMode=Boolean
  Logical Operator2 : Logic  Operator=OR  AllPortsSameDT=off  OutDataTypeMode=Boolean  SampleTime=.001
  Memory : Memory  Orientation=left
  Relational Operator : RelationalOperator  Operator=>  LogicOutDataTypeMode=Boolean
  Sum : Sum  Inputs=-+
  Time : Constant  Value=Time
  Out1 : Outport
  wires:
  Clock/1 -> Enabled Subsystem/1(In1), Sum/2
  Enabled Subsystem/1(Out1) -> Sum/1
  Sum/1 -> Compare To Zero/1, Relational Operator/1
  Time/1 -> Relational Operator/2
  Compare To Zero/1 -> Logical Operator/1
  Relational Operator/1 -> Logical Operator/2
  Logical Operator1/1 -> Enabled Subsystem/Enable
  Logical Operator/1 -> Out1/1, Memory/1
  In1/1 -> Logical Operator2/2
  Logical Operator2/1 -> Logical Operator1/1
  Memory/1 -> Logical Operator2/1

== system limblab/BehaviorOutputSystem/RewardSbs/Schmidt1/Enabled Subsystem ==
  In1 : Inport
  Enable : EnablePort
  Out1 : Outport
  wires:
  In1/1 -> Out1/1

== system limblab/RobotInputSystem/XY Position Subsystem/For Iterator Subsystem/While Iterator Subsystem ==
  Start Time : Inport
  Reward : Inport  Port=2
  Compare To Constant : simulink/Logic and Bit Operations/Compare To Constant  SystemSampleTime=-1  relop=<=  const=200  LogicOutDataTypeMode=boolean
  Compare To Constant1 : simulink/Logic and Bit Operations/Compare To Constant  SystemSampleTime=-1  relop=>  const=100  LogicOutDataTypeMode=boolean  ZeroCross=off
  Constant : Constant
  Constant1 : Constant  Value=0
  "PCI-6025E " : xpcnilib/Digital Output/PCI-6025E DO  channel=[1 2]  reset=[1]  initValue=[0]  sampletime=-1  slot=-1
  ScaleTouSec : Gain  Gain=.838
  Subtract : Sum  Inputs=+-  OutScaling=2^-10
  Switch : Switch  Criteria=u2 ~= 0
  While Iterator : WhileIterator  MaxIters=-1  WhileBlockType=do-while
  "xPC Target  Time " : xpclib/Misc./xPC Target  Time   ts=-1
  wires:
  "xPC Target  Time "/1 -> Subtract/1
  Start Time/1 -> Subtract/2
  Subtract/1 -> ScaleTouSec/1
  Compare To Constant/1 -> While Iterator/1
  ScaleTouSec/1 -> Compare To Constant/1, Compare To Constant1/1
  Compare To Constant1/1 -> Switch/2
  Constant/1 -> Switch/1
  Constant1/1 -> Switch/3
  Switch/1 -> "PCI-6025E "/1
  Reward/1 -> "PCI-6025E "/2

== system limblab/RobotOutputSystem/Motor Control/Schmidt/Enabled Subsystem ==
  In1 : Inport
  Enable : EnablePort
  Out1 : Outport
  wires:
  In1/1 -> Out1/1

== system limblab/RobotOutputSystem/Recentering Subsystem/Schmidt1/Enabled Subsystem ==
  In1 : Inport
  Enable : EnablePort
  Out1 : Outport
  wires:
  In1/1 -> Out1/1

== system limblab/RobotOutputSystem/Recentering Subsystem/Schmidt2/Enabled Subsystem ==
  In1 : Inport
  Enable : EnablePort
  Out1 : Outport
  wires:
  In1/1 -> Out1/1

== system limblab/RobotOutputSystem/Recentering Subsystem/Schmidt3/Enabled Subsystem ==
  In1 : Inport
  Enable : EnablePort
  Out1 : Outport
  wires:
  In1/1 -> Out1/1
